simulink library "Window"  (Simulink 8.2)
settings: Solver=ode45  StartTime=0.0  StopTime=10.0  RelTol=1e-3
undefined symbols (not defined in the file): frame, g, pos, t0, tau, windowsize
libraries: carnot x3
settings Model: Creator=lena.frank  LastModifiedBy=drhf

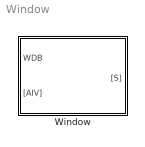
== system Window ==
  Window : Subsystem  mask(outer wall){wallsize=windowsize, frame=frame, pos=pos, t0=t0, d=[0.03 0.03], cond=[.81 .81], cwall=[.28 .28]*3600, rho=[2500 2500], misc=[0.2 0.1 1 1], gvalue=g, tau=tau, dactive=[0.01 0.05]}
      mask prompts: wallsize "size of window [m] [height width]"; frame "part of frame of the surface (0..1)"; pos "azimut (0=south, east = -90)"; t0 "initial temperature [degree centigrade]"; d "thickness of nodes [m] (vector)"; cond "conductivity of nodes [W/(m*K)] (vector)"; cwall "capacity of nodes [J/(kg*K)] (vector)"; rho "density [kg/m^3]"; misc "[reflection_ground absorption_out emission_out emission_in]"; gvalue "energy transmission of window (0..1)"; tau "time-constant of window [s]"; dactive "depth of active layer [m] (-1, if none; start at outside)"
      mask help:
      | This is the model of a window of a house.
      | first element of the vector = layer to surrounding
      | last element of the vector = layer to room
      mask init:
      | nodes = length(d);
      | numlayer = nodes;
      | position = [90  pos  0];
      | 
      | h = wallsize(1);
      | w = wallsize(2);
      | %für Variablen in shaderad
      | reflectground = min(0, max(1, misc(1)));
      | 
      | wallangle = position(1);
      | wallazimut = position(2);
      | wallheight=h;
      | wallwidth=w;
      | wallsurface = h*w;
      | 
      | absorption_out = misc(2);
      | emission_out = misc(3);
      | emission_in = misc(4);
      mask Help: web(fullfile(path_carnot('help'),'Window.html'),'-helpbrowser')

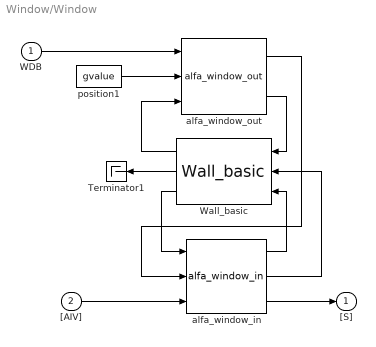
== system Window/Window ==
  WDB : Inport
  "[AIV]" : Inport  Port=2
  Terminator1 : Terminator
  Wall_basic : carnot/Basic/Thermal_Models/Wall_basic
  alfa_window_in : carnot/Load/Houses/heat_transfer/alfa_window_in
  alfa_window_out : carnot/Load/Houses/heat_transfer/alfa_window_out
  position1 : Constant  Value=gvalue
  "[S]" : Outport
  wires:
  alfa_window_in/2 -> Wall_basic/2
  Wall_basic/3 -> alfa_window_in/1
  alfa_window_out/2 -> Wall_basic/1
  Wall_basic/2 -> Terminator1/1
  alfa_window_out/1 -> alfa_window_in/2
  WDB/1 -> alfa_window_out/1
  alfa_window_in/3 -> "[S]"/1
  alfa_window_in/1 -> Wall_basic/3
  "[AIV]"/1 -> alfa_window_in/3
  position1/1 -> alfa_window_out/2
  Wall_basic/1 -> alfa_window_out/3
